simulink model "homework1_1"  (R2023a)
settings: Solver=VariableStepAuto  StartTime=0.0  StopTime=10.0  RelTol=1e-3
libraries: spsMultimeterLib x4, spsControlledVoltageSourceLib x1, spsSeriesRLCBranchLib x1, spsUniversalBridgeLib x1, spspowerguiLib x1
settings Model: Creator=zou20  LastModifiedBy=zou20

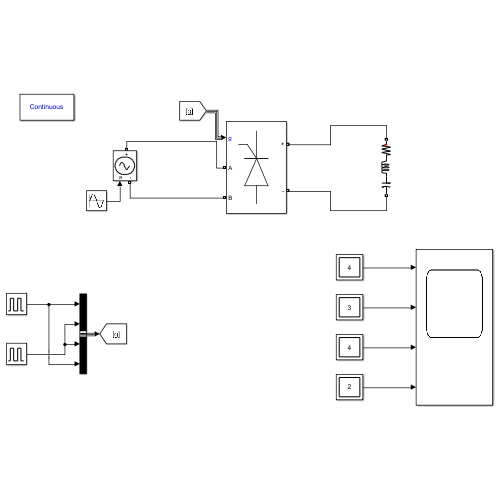
[thumbnail: Simulink's stored preview of the top-level diagram]
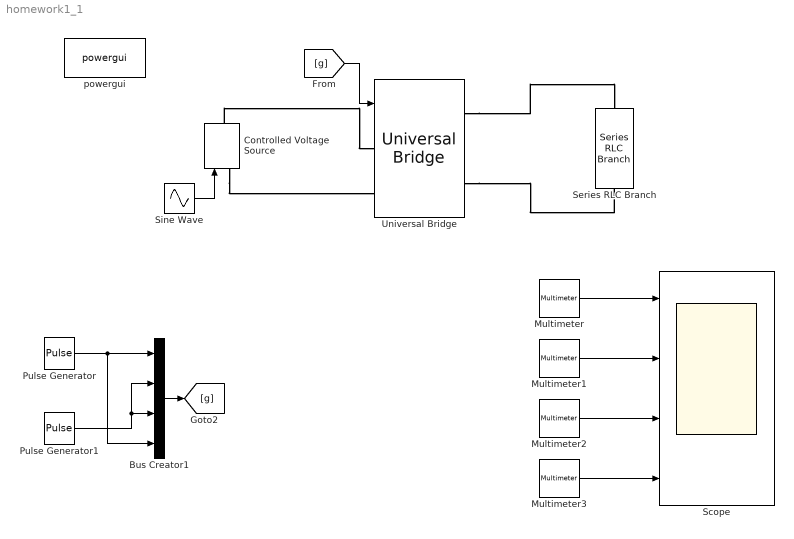
== system homework1_1 ==
  Bus Creator1 : BusCreator  Inputs=4
  Controlled Voltage Source : spsControlledVoltageSourceLib/Controlled Voltage Source  Initialize=on  Source_Type=AC  Amplitude=0  Phase=0  Frequency=50  Measurements=Voltage
  Multimeter : spsMultimeterLib/Multimeter  L=13  sel=[10 11 12 13]  yselected={}  Gain=[1 1 1 1]  OutputType=Complex  PlotAtSimulationStop=off  PhasorSimulation=off
  Multimeter1 : spsMultimeterLib/Multimeter  L=13  sel=[6 7 8]  yselected={}  Gain=[1 1 1]  OutputType=Complex  PlotAtSimulationStop=off  PhasorSimulation=off
  Multimeter2 : spsMultimeterLib/Multimeter  L=13  sel=[2 3 4 5]  yselected={}  Gain=[1 1 1 1]  OutputType=Complex  PlotAtSimulationStop=off  PhasorSimulation=off
  Multimeter3 : spsMultimeterLib/Multimeter  L=13  sel=[1 9]  yselected={}  Gain=[1 1]  OutputType=Complex  PlotAtSimulationStop=off  PhasorSimulation=off
  Pulse Generator : DiscretePulseGenerator  PulseType=Time based  Amplitude=3  Period=0.02  PulseWidth=10
  Pulse Generator1 : DiscretePulseGenerator  PulseType=Time based  Amplitude=3  Period=0.02  PulseWidth=10  PhaseDelay=0.01
  Scope : Scope  NumInputPorts=4
  Series RLC Branch : spsSeriesRLCBranchLib/Series RLC Branch  LConnTagsString=__new0  RConnTagsString=__new0  BranchType=RLC  Resistance=1000  Inductance=0  SetiL0=off  InitialCurrent=0  Capacitance=0  Setx0=off  InitialVoltage=0  Measurements=Branch voltage and current
  Sine Wave : Sin  Amplitude=110*sqrt(2)  Frequency=2*pi*50  SampleTime=0
  Universal Bridge : spsUniversalBridgeLib/Universal Bridge  Arms=2  SnubberResistance=1e5  SnubberCapacitance=inf  Device=Thyristors  Ron=1e-3  Lon=0  ForwardVoltages="[  0  0  ]"  ForwardVoltage=0  GTOparameters=[ 10e-6 , 20e-6 ]  IGBTparameters=[ 1e-6 , 2e-6 ]  Measurements=All voltages and currents  Measurements_2=None  converterType=Rectifier
  powergui : spspowerguiLib/powergui  Priority=1  SimulationMode=Continuous  SampleTime=50e-6  frequency=60  Iterations=50  frequencyindice=50  Pbase=100e6  ErrMax=1e-4  UnitsV=kV  UnitsW=MW  buscounter=0  FunctionMessages=off  echomessages=off  EnableUseOfTLC=off  CurrentSourceSwitches=off  DisableSnubberDevices=off  DisableRonSwitches=off  DisableVfSwitches=off  DisplayEquations=off  AutomaticDiscreteSolvers=off  SolverType=Tustin/Backward Euler (TBE)  Interpol=off  ExternalGateDelay=off  methode=off  Ts=100  x0status=blocks  SPID=on  SwTol=0  HookPort=off  NonlinearTolerance=1e-4  nMaxIteration=100  ContinueOnMaxIteration=off  RestoreLinks=warning  ResistiveCurrentMeasurement=off  Frange=[0:2:500]  Ylog=off  Xlog=on  ShowGrid=off  save=off  variable=ZData  structure=0  ZoomFFT=off  StartTime=0.0  cycles=1  DisplayStyle=1  fundamental=60  FreqAxis=off  MaxFrequency=1000  frequencyindicesteady=1  RmsSteady=1  display=off
  wires:
  Pulse Generator1/1 -> Bus Creator1/3, Bus Creator1/2
  Pulse Generator/1 -> Bus Creator1/4, Bus Creator1/1
  Bus Creator1/1 -> [g]
  [g] -> Universal Bridge/1
  Sine Wave/1 -> Controlled Voltage Source/1
  Multimeter/1 -> Scope/1
  Multimeter1/1 -> Scope/2
  Multimeter2/1 -> Scope/3
  Multimeter3/1 -> Scope/4
  connections:
  Controlled Voltage Source/LConn1 -- Universal Bridge/LConn2
  Controlled Voltage Source/RConn1 -- Universal Bridge/LConn1
  Universal Bridge/RConn1 -- Series RLC Branch/LConn1
  Universal Bridge/RConn2 -- Series RLC Branch/RConn1
